simulink model "exemple3"  (R2021a)
settings: Solver=VariableStepAuto  StartTime=0.0  StopTime=20  RelTol=1e-3
libraries: dspsrcs4 x2, dspswit3 x2, commfilt2 x2, simulink x1, dspsigops x1
settings Model: Creator=sebastienroy  LastModifiedBy=sebastienroy
settings SolverCC: AlgebraicLoopSolver=TrustRegion
settings DebuggingCC: SFMachineParentedDataDiag=warning

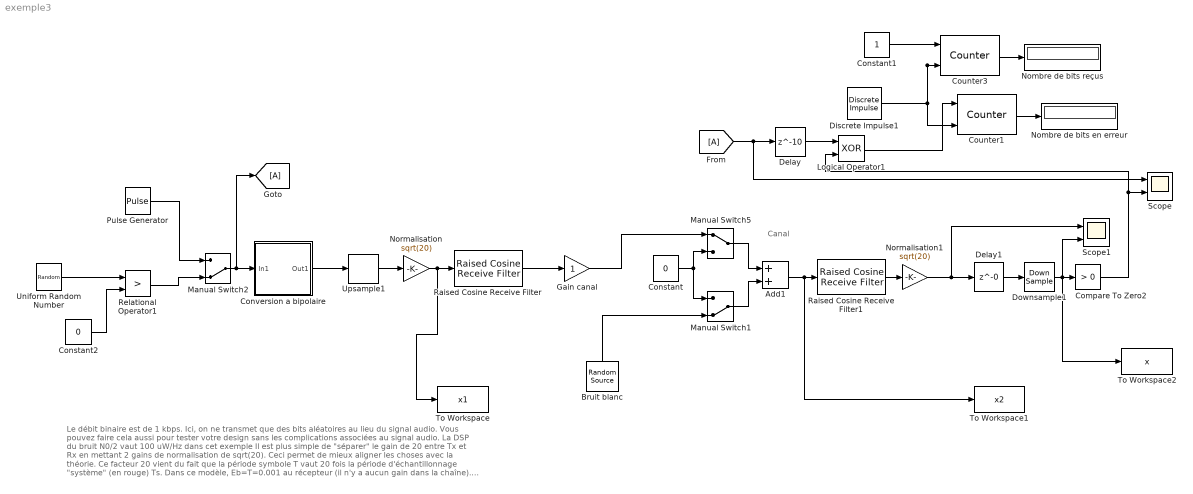
== system exemple3 ==
  note: Le débit binaire est de 1 kbps. Ici, on ne transmet que des bits aléatoires au lieu du signal audio. Vous pouvez faire cela aussi pour tester votre design sans les complications associées au signal audio.
      |
      | La DSP du bruit N0/2 vaut 100 uW/Hz dans cet exemple
      |
      | Il est plus simple de "séparer" le gain de 20 entre Tx et Rx en mettant
      | 2 gains de normalisation de sqrt(20). Ceci permet de mieux aligner les
      | choses avec la théorie.
      |
      | Ce facteur 20 vient du fait que la période symbole T vaut 20 fois la période d'échantillonnage "système" (en rouge) Ts.
      |
      | Dans ce modèle, Eb=T=0.001 au récepteur (il n'y a aucun gain dans la chaîne). Ceci fait qu'en théorie, Pb=Q(sqrt(10))=Q(3.162)=7.9 x 10^-4.
      |
      | Le compteur d'erreur confirme ce taux d'erreur en simulation.
      |
      | NOTE: Vous devez utiliser le bloc "Square Root Receive Filter" aux deux bouts. Éviter le bloc "Square Root Transmit Filter," car on veut que l'interpolation se fasse explicitement à l'exztérieur du bloc.
  note: Canal
  Add1 : Sum
  "Bruit blanc " : dspsrcs4/Random Source  SrcType=Gaussian  NormMethod=Ziggurat  CltLength=12  MinVal=0  MaxVal=1  MeanVal=0  VarVal=2  RepMode=Not repeatable  rawSeed=1  IsInherit=on  SampMode=Discrete  SampTime=1  SampFrame=1  DataType=Double  OutComplex=Real  OutputFrames=on
  Compare To Zero2 : simulink/Logic and Bit Operations/Compare To Zero  relop=>  OutDataTypeStr=boolean
  Constant : Constant  Value=0
  Constant1 : Constant  SampleTime=1/1000
  Constant2 : Constant  Value=0
  Conversion a bipolaire : Subsystem
  Counter1 : dspswit3/Counter  Direction=Up  CountEvent=Non-zero sample  CounterSize=32 bits  MaxCount=255  InitialCount=0  Output=Count  HitValue=32  ResetInput=on  SamplesPerFrame=1  Ts=1/10000  CntDtype=uint32  HitDtype=Logical
  Counter3 : dspswit3/Counter  Direction=Up  CountEvent=Non-zero sample  CounterSize=32 bits  MaxCount=255  InitialCount=0  Output=Count  HitValue=32  ResetInput=on  SamplesPerFrame=1  Ts=1/10000  CntDtype=uint32  HitDtype=Logical
  Delay : Delay  DelayLength=10  InitialCondition=0
  Delay1 : Delay  DelayLength=0  InitialCondition=0
  Discrete Impulse1 : dspsrcs4/Discrete  Impulse  Delay=10  SampleTime=1/1000  FrameSample=1  OutputFrames=on  dataType=double  isSigned=on  wordLen=16  udDataType=sfix(16)  fracBitsMode=Best precision  numFracBits=15  OutDataTypeStr=double  LastOutDataTypeStr=double
  Downsample1 : DownSample  N=20  RateOptions=Allow multirate processing
  Gain canal : Gain
  Logical Operator1 : Logic  Operator=XOR  AllPortsSameDT=off  OutDataTypeStr=boolean
  Manual Switch1 : ManualSwitch  CurrentSetting=0
  Manual Switch2 : ManualSwitch  CurrentSetting=0
  Manual Switch5 : ManualSwitch
  Nombre de bits en erreur : Display
  Nombre de bits reçus : Display
  Normalisation : Gain  Gain=sqrt(20)
  Normalisation1 : Gain  Gain=sqrt(20)
  Pulse Generator : DiscretePulseGenerator  SampleTime=1/1000
  Raised Cosine Receive Filter : commfilt2/Raised Cosine Receive Filter  filtType=Square root  R=0.2  filtSpan=10  N=20  downFactor=1  downOffset=0  filterGain=1  RateOptions=Allow multirate processing  framing=Mute  checkCoeff=on  variableName=rcRxFilt  currentFiltSpan=10  D=5  inputOffset=0  sampMode=Mute  saveAsFlag=0  rateMode=Downsampling  checkGain=Normalized  launchFVT=on  roundingMode=Floor  overflowMode=off  coeffDataTypeStr=Inherit: Same word length as input  coeffMin=[]  coeffMax=[]  coeffLastDataTypeStr=Inherit: Same word length as input  accumDataTypeStr=Inherit: Same as product output  accumLastDataTypeStr=Inherit: Same as product output  outputDataTypeStr=Inherit: Same as accumulator  outputMin=[]  outputMax=[]  outputLastDataTypeStr=Inherit: Same as accumulator
  Raised Cosine Receive Filter1 : commfilt2/Raised Cosine Receive Filter  filtType=Square root  R=0.2  filtSpan=10  N=20  downFactor=1  downOffset=0  filterGain=1  RateOptions=Allow multirate processing  framing=Mute  checkCoeff=on  variableName=rcRxFilt1  currentFiltSpan=10  D=5  inputOffset=0  sampMode=Mute  saveAsFlag=0  rateMode=Downsampling  checkGain=Normalized  launchFVT=on  roundingMode=Floor  overflowMode=off  coeffDataTypeStr=Inherit: Same word length as input  coeffMin=[]  coeffMax=[]  coeffLastDataTypeStr=Inherit: Same word length as input  accumDataTypeStr=Inherit: Same as product output  accumLastDataTypeStr=Inherit: Same as product output  outputDataTypeStr=Inherit: Same as accumulator  outputMin=[]  outputMax=[]  outputLastDataTypeStr=Inherit: Same as accumulator
  Relational Operator1 : RelationalOperator  Operator=>  OutDataTypeStr=boolean  RndMeth=Nearest
  Scope : Scope  NumInputPorts=2
  Scope1 : Scope  NumInputPorts=2
  To Workspace : ToWorkspace  VariableName=x1  SampleTime=-1
      settings: Save2DSignal=2-D array (concatenate along first dimension)
  To Workspace1 : ToWorkspace  VariableName=x2  SampleTime=-1
      settings: Save2DSignal=2-D array (concatenate along first dimension)
  To Workspace2 : ToWorkspace  VariableName=x  SampleTime=-1
      settings: Save2DSignal=2-D array (concatenate along first dimension)
  Uniform Random Number : UniformRandomNumber  Seed=3  SampleTime=1/1000
  Upsample1 : dspsigops/Upsample  N=20  phase=0  RateOptions=Allow multirate processing  ic=0  mode=Unused parameter value
  wires:
  Raised Cosine Receive Filter/1 -> Gain canal/1
  Normalisation/1 -> Raised Cosine Receive Filter/1, To Workspace/1
  Upsample1/1 -> Normalisation/1
  Constant2/1 -> Relational Operator1/2
  Uniform Random Number/1 -> Relational Operator1/1
  Manual Switch5/1 -> Add1/1
  Manual Switch1/1 -> Add1/2
  "Bruit blanc "/1 -> Manual Switch1/2
  Constant/1 -> Manual Switch5/2, Manual Switch1/1
  Raised Cosine Receive Filter1/1 -> Normalisation1/1
  Downsample1/1 -> To Workspace2/1, Scope1/2, Compare To Zero2/1
  Delay1/1 -> Downsample1/1
  Conversion a bipolaire/1(Out1) -> Upsample1/1
  Relational Operator1/1 -> Manual Switch2/2
  Pulse Generator/1 -> Manual Switch2/1
  Manual Switch2/1 -> [A], Conversion a bipolaire/1(In1)
  Gain canal/1 -> Manual Switch5/1
  Add1/1 -> To Workspace1/1, Raised Cosine Receive Filter1/1
  Normalisation1/1 -> Scope1/1, Delay1/1
  Constant1/1 -> Counter3/1
  Discrete Impulse1/1 -> Counter3/2, Counter1/2
  Counter1/1 -> Nombre de bits en erreur/1
  Counter3/1 -> Nombre de bits reçus/1
  Compare To Zero2/1 -> Logical Operator1/2, Scope/2
  Delay/1 -> Logical Operator1/1
  Logical Operator1/1 -> Counter1/1
  [A] -> Scope/1, Delay/1

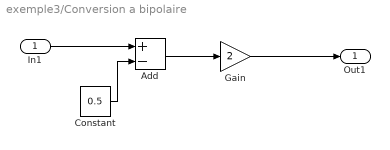
== system exemple3/Conversion a bipolaire ==
  In1 : Inport
  Add : Sum  Inputs=+-
  Constant : Constant  Value=0.5
  Gain : Gain  Gain=2
  Out1 : Outport  VectorParamsAs1DForOutWhenUnconnected=off
  wires:
  In1/1 -> Add/1
  Add/1 -> Gain/1
  Constant/1 -> Add/2
  Gain/1 -> Out1/1
